simulink model "ASmodelViskozni"  (R2021a)
settings: Solver=VariableStepAuto  StartTime=0.0  StopTime=10.0  RelTol=1e-3
values from neighbouring files (symbols this model uses):
  J = 0.1    [DemoParam.mat]    (also in DemoParametry.mat; Mereni.m = 1/(dwdt*Mz); TeorParam.mat = 0.363889989323)
  Lh = 0.3    [DemoParam.mat]    (also in DemoParametry.mat; TeorParam.m = ((U0f)^2*3)/(2*pi*50*sqrt((3*S0_1f)^2-(3*P0_1f)^2)); TeorParam.mat = 0.131626294416; TeorParamPokus.m)
  pp = 1    [DemoParam.mat]    (also in DemoParametry.mat; TeorParam.m = 2; TeorParam.mat = 2; TeorParamPokus.m)
  Umax = sqrt(2)*U1    [ParametryAS.m]
undefined symbols (not defined in the file or in its folder): Lr, Ls, Rr, Rs
settings Model: Creator=vojta  LastModifiedBy=vojta

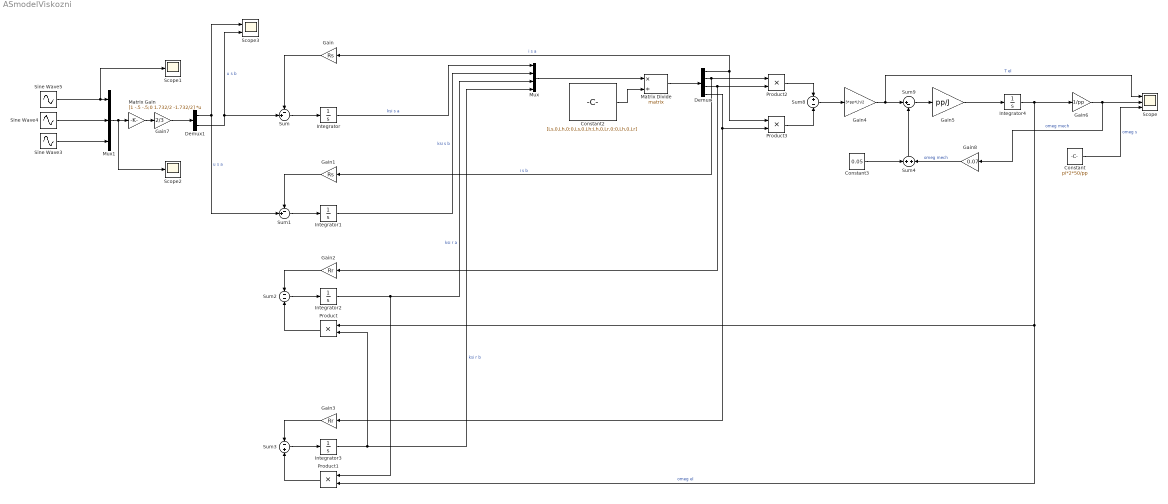
== system ASmodelViskozni ==
  Constant : Constant  Value=pi*2*50/pp
  Constant2 : Constant  Value=[Ls,0,Lh,0;0,Ls,0,Lh;Lh,0,Lr,0;0,Lh,0,Lr]
  Constant3 : Constant  Value=0.05
  Demux : Demux
  Demux1 : Demux  Outputs=2
      settings: DisplayOption=none
  Gain : Gain  Gain=Rs
  Gain1 : Gain  Gain=Rs
  Gain2 : Gain  Gain=Rr
  Gain3 : Gain  Gain=Rr
  Gain4 : Gain  Gain=3*pp*Lh/2
  Gain5 : Gain  Gain=pp/J
  Gain6 : Gain  Gain=1/pp
  Gain7 : Gain  Gain=2/3  SaturateOnIntegerOverflow=on  OutDataTypeStr=Inherit: Same as input  ParamDataTypeStr=Inherit: Same as input
  Gain8 : Gain  Gain=0.07
  Integrator{,1..4} (5 alike) : Integrator
  Matrix Gain : Gain  Gain=[1 -.5 -.5;0 1.732/2 -1.732/2]  Multiplication=Matrix(K*u)  SaturateOnIntegerOverflow=on  OutDataTypeStr=Inherit: Same as input  ParamDataTypeStr=Inherit: Same as input
  Matrix Divide : Product  Inputs=*/  Multiplication=Matrix(*)
  Mux : Mux
  Mux1 : Mux  Inputs=3
  Product{,1..3} (4 alike) : Product
  Scope : Scope  NumInputPorts=3
  Scope1 : Scope
  Scope2 : Scope
  Scope3 : Scope  NumInputPorts=2
  Sine Wave3 : Sin  Amplitude=Umax  Frequency=100*pi  Phase=-2*pi/3
  Sine Wave4 : Sin  Amplitude=Umax  Frequency=100*pi  Phase=2*pi/3
  Sine Wave5 : Sin  Amplitude=Umax  Frequency=100*pi
  Sum : Sum  Inputs=-+|
  Sum1 : Sum  Inputs=-+|
  Sum2 : Sum  Inputs=--
  Sum3 : Sum  Inputs=-+
  Sum4 : Sum
  Sum8 : Sum  Inputs=+-
  Sum9 : Sum  Inputs=|+-
  wires:
  Sum/1 -> Integrator/1
  Sum1/1 -> Integrator1/1
  Sum2/1 -> Integrator2/1
  Sum3/1 -> Integrator3/1
  Integrator/1 -> Mux/1  "ksi s a"
  Integrator1/1 -> Mux/2  "ksi s b"
  Integrator2/1 -> Product1/1, Mux/3  "ksi r a"
  Integrator3/1 -> Product/2, Mux/4  "ksi r b"
  Demux1/1 -> Sum1/2, Scope3/1  "u s a"
  Demux1/2 -> Sum/2, Scope3/2  "u s b"
  Gain/1 -> Sum/1
  Gain1/1 -> Sum1/1
  Constant2/1 -> Matrix Divide/2
  Mux/1 -> Matrix Divide/1
  Matrix Divide/1 -> Demux/1
  Demux/1 -> Product3/1, Gain/1  "i s a"
  Demux/2 -> Product2/1, Gain1/1  "i s b"
  Gain2/1 -> Sum2/1
  Demux/3 -> Gain2/1, Product2/2
  Product/1 -> Sum2/2
  Gain3/1 -> Sum3/1
  Demux/4 -> Gain3/1, Product3/2
  Product1/1 -> Sum3/2
  Sum8/1 -> Gain4/1
  Product2/1 -> Sum8/1
  Product3/1 -> Sum8/2
  Sum9/1 -> Gain5/1
  Gain5/1 -> Integrator4/1
  Integrator4/1 -> Product1/2, Product/1, Gain6/1  "omeg el"
  Gain6/1 -> Gain8/1, Scope/2  "omeg mech"
  Gain4/1 -> Scope/1, Sum9/1  "T el"
  Mux1/1 -> Scope2/1, Matrix Gain/1
  Gain7/1 -> Demux1/1
  Sine Wave3/1 -> Mux1/3
  Sine Wave4/1 -> Mux1/2
  Matrix Gain/1 -> Gain7/1
  Sine Wave5/1 -> Scope1/1, Mux1/1
  Constant/1 -> Scope/3  "omeg s"
  Constant3/1 -> Sum4/1
  Sum4/1 -> Sum9/2
  Gain8/1 -> Sum4/2  "omeg mech"
